simulink model "car_model_FIXED"  (R2022b)
settings: Solver=VariableStepAuto  StartTime=0.0  StopTime=60  RelTol=1e-3
values from neighbouring files (symbols this model uses):
  ABS_MAX_TORQUE = [25 25 25 25]    [Startup.m]
  ABS_MAX_TRQ_CMD = dot(ABS_MAX_TORQUE, MOTOR_ENABLE)    [Startup.m]
  ABS_MIN_TORQUE = [0.01 0.01 0.01 0.01]    [Startup.m]
  acc_IC = 0    [Startup.m]
  ACCELERATION_MAX = 30    [Startup.m]
  ang_IC = 0    [Startup.m]
  ang_vel_IC = 0    [Startup.m]
  ax = Reference_Signals.Chassis_Acceleration_VNED.ax.Data(:)    [Simulation_Data_Parse.m]    (also in Vehicle_Sim_Parse.m)
  ay = Reference_Signals.Chassis_Acceleration_VNED.ay.Data(:)    [Simulation_Data_Parse.m]    (also in Vehicle_Sim_Parse.m)
  az = Reference_Signals.Chassis_Acceleration_VNED.az.Data(:)    [Simulation_Data_Parse.m]    (also in Vehicle_Sim_Parse.m)
  battery_current_IC = 0    [Startup.m]
  BATTERY_CURRENT_MAX = 140    [Startup.m]
  BATTERY_CURRENT_MIN = 0    [Startup.m]
  battery_FT_IC = 300    [Startup.m]
  battery_T_IC = 300    [Startup.m]
  BATTERY_TEMPERATURE_MAX = 60    [Startup.m]
  BATTERY_TEMPERATURE_MIN = 0    [Startup.m]
  battery_voltage_IC = Ns*max(Em)    [Startup.m]
  BATTERY_VOLTAGE_MAX = 340    [Startup.m]
  BATTERY_VOLTAGE_MIN = 60    [Startup.m]
  Brake_Pressure_IC = 1    [Startup.m]
  ccl_IC = 0    [Startup.m]
  CENTER_STEER_ANGLE_MAX = 130    [Startup.m]
  covarience_matrix_IC = Simulink.Parameter(eye(28)./1000)    [Startup.m]
  dcl_IC = 140    [Startup.m]
  DCL_MAX = 130    [Startup.m]
  DCL_MIN = 0    [Startup.m]
  driver_t = 0.015    [Startup.m]
  fusion_t = Simulink.Parameter(0.01)    [Startup.m]
  fusion_t_sim = fusion_t.copy    [Startup.m]
  Fz_IC = m_all*g/4    [Startup.m]
  g = 9.81    [Startup.m]
  gps_hz = 0.01    [Startup.m]
  gps_ratio = Simulink.Parameter(gps_hz / imu_hz.Value)    [Startup.m]
  imu_hz = fusion_t.copy    [Startup.m]
  location_lla_IC = Simulink.Parameter([40.437675, -86.943750, 200])    [Startup.m]
  MAG_MAX = 200    [Startup.m]
  Max_Brake_Pressure = 10^8    (= 100000000)    [Startup.m]
  Max_Driver_Input = 1    [Startup.m]
  MAX_DTHETA_DRIVER = 360    [Startup.m]
  MAX_STEERING_ADJUST = 15    [Startup.m]
  Min_Brake_Pressure = 1    [Startup.m]
  Min_Driver_Input = 0    [Startup.m]
  motor_current_IC = 0    [Startup.m]
  MOTOR_CURRENT_MAX = 70    [Startup.m]
  MOTOR_CURRENT_MIN = 0    [Startup.m]
  MOTOR_ENABLE = [0 0 1 1]    [Startup.m]
  motor_FT_IC = 300    [Startup.m]
  motor_T_IC = 300    [Startup.m]
  MOTOR_TEMPERATURE_MAX = 100    [Startup.m]
  MOTOR_TEMPERATURE_MIN = 0    [Startup.m]
  motor_voltage_IC = 332    [Startup.m]
  MOTOR_VOLTAGE_MAX = 340    [Startup.m]
  MOTOR_VOLTAGE_MIN = 90    [Startup.m]
  omega_IC = 0    [Startup.m]
  OMEGA_MAX = 150    [Startup.m]
  OMEGA_MIN = 0    [Startup.m]
  ORIENTATION_MAX = 360    [Startup.m]
  pos_IC = 0    [Startup.m]
  POS_MAX = 300    [Startup.m]
  rho = 1.225    [Startup.m]
  selected_maxvm = MIN_TRACK_DATA.(event_names(10))    [Startup.m]
  selected_sweep = ALL_SWEEP_DATA.(sweep_names(1))    [Startup.m]
  selected_track = ALL_TRACK_DATA.(event_names(10))    [Startup.m]
  shock_length_IC = 0.1    [Startup.m]
  SHOCK_LENGTH_MAX = 0.25    [Startup.m]
  SHOCK_LENGTH_MIN = 0    [Startup.m]
  state_IC = zeros(28,1)    [Startup.m]
  theta_IC = 0    [Startup.m]
  TRACTION_ENABLE = 0    [Startup.m]
  TVS_ENABLE = 0    [Startup.m]
  tvs_t = 0.015    [Startup.m]
  tvs_t_sim = tvs_t    (= 0.015)    [Startup.m]
  Tx_I = 0    [Startup.m]
  vel_IC = [0 0 0]    [Startup.m]
  VELOCITY_MAX = 30    [Startup.m]
  X = Reference_Signals.Chassis_Position.X.Data(:)    [Simulation_Data_Parse.m]    (also in Vehicle_Sim_Parse.m = Chassis_Signals.InertFrm.Cg.Disp.X.Data(:))
  Y = Reference_Signals.Chassis_Position.Y.Data(:)    [Simulation_Data_Parse.m]    (also in Vehicle_Sim_Parse.m = Chassis_Signals.InertFrm.Cg.Disp.Y.Data(:))
  YAW_ENABLE = 1    [Startup.m]
  YAW_MAX = 2.5    [Startup.m]
undefined symbols (not defined in the file or in its folder): ActSuspDutyCycle, Aeq_left, Aeq_right, alpha_error, ang_acc_hystersesis, area_air, axb, br, brake_bias, covA, covG, covM, covP, covV, CURRENT_BUFFER, cy_sweep, dB, deadband_angle, dIndex, DiscIntNeverNeededParam, dt_OFF, dt_ON, dTx, dx, dZ, efficiency_grid, F0z, forward_look_straight, forward_look_turn, Fz_sweep, GAIN_ABS, gearbox_efficiency, gr, I, I_Driver, IMU_accel, IMU_gyro, IMU_mag, IMUNED2VNED, indicies, IYY, kx_sweep, l, lambda_star, low_V_SA, lr, m_all, m_body, m_unsprung, MAGNED2VNED, MAX_I_Driver, max_yaw, min_velocity_regen, motorControllerCurve, motorTempCurve, motorTempX, mu_star, mx_sweep, my_sweep, noise_state ... (+40)
libraries: fl_lib x82, nesl_utility x32, vehdynlibtire x10, vehdynlibsuspension x8, simulink x5, autolibutils x5, sharedtransform x5, sdl_lib x4, EngineCoolingComponents_lib x4, slpidlib x3, SimscapeFluids_lib x3, shared6dof x2
(part 5 of 14)

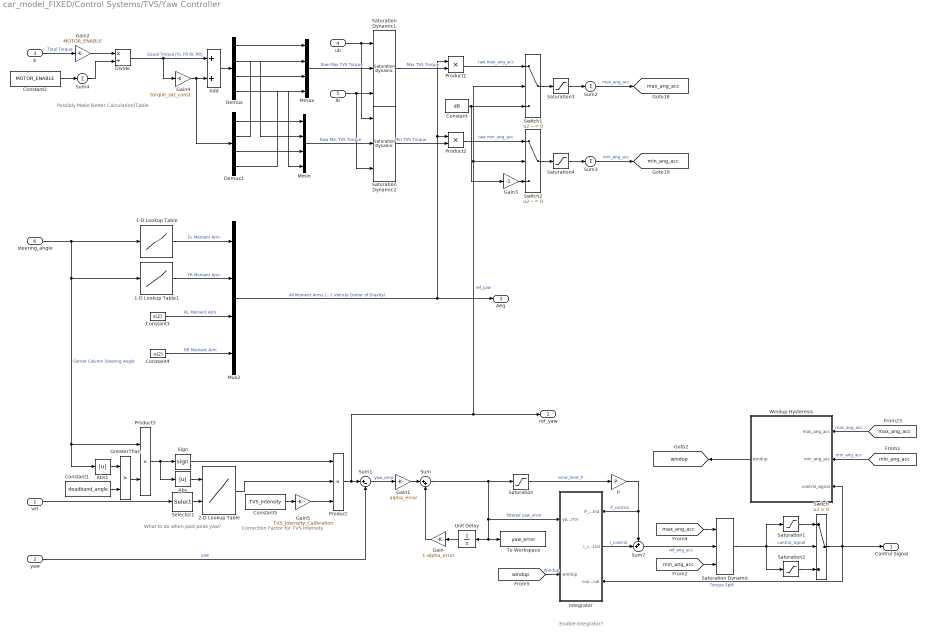
== system car_model_FIXED/Control Systems/TVS/Yaw Controller ==
  note: Correction Factor for TVS Intensity
  note: Enable Integrator?
  note: What to do when past peak yaw?
  note: Possibly Make Better Calculation/Table
  vel : Inport
  yaw : Inport  Port=2  OutDataTypeStr=double  LockScale=on
  b : Inport  Port=3
  ub : Inport  Port=4
  lb : Inport  Port=5
  steering_angle : Inport  Port=6
  1-D Lookup Table : Lookup_n-D  NumberOfTableDimensions=1  BreakpointsForDimension1=theta_sweep  Table=Aeq_left  ExtrapMethod=Clip  InternalRulePriority=Speed  RndMeth=Simplest
  1-D Lookup Table1 : Lookup_n-D  NumberOfTableDimensions=1  BreakpointsForDimension1=theta_sweep  Table=Aeq_right  ExtrapMethod=Clip  InternalRulePriority=Speed  RndMeth=Simplest
  2-D Lookup Table : Lookup_n-D  BreakpointsForDimension1=steering_sweep  BreakpointsForDimension2=velocity_sweep  Table=yaw_rate  ExtrapMethod=Clip  InternalRulePriority=Speed  RndMeth=Simplest
      settings: InputPortMap=u0,u1
  Abs : Abs  SaturateOnIntegerOverflow=off
  Abs1 : Abs  SaturateOnIntegerOverflow=off
  Add : Sum
  Constant : Constant  Value=dB  OutDataTypeStr=Inherit: Inherit via back propagation
  Constant1 : Constant  Value=deadband_angle
  Constant2 : Constant  Value=MOTOR_ENABLE
  Constant3 : Constant  Value=s(2)  OutDataTypeStr=Inherit: Inherit via back propagation
  Constant4 : Constant  Value=-s(2)  OutDataTypeStr=Inherit: Inherit via back propagation
  Constant5 : Constant  Value=TVS_Intensity
  Demux : Demux
  Demux1 : Demux
  Divide : Product  Inputs=*/
  Gain : Gain  Gain=1-alpha_error
  Gain1 : Gain  Gain=alpha_error
  Gain2 : Gain  Gain=MOTOR_ENABLE
  Gain3 : Gain  Gain=-1
  Gain4 : Gain  Gain=torque_sat_const
  Gain5 : Gain  Gain=TVS_Intensity_Calibration
  GreaterThan : RelationalOperator  Operator=>  OutDataTypeStr=boolean  RndMeth=Simplest  InputSameDT=off
  Integrator : Subsystem
      settings: PortSchema="{\"entries\":[{\"content\":{\"sides\":[{\"content\":{\"connectorIds\":[\"In1\",\"In2\"]},\"type\":\"ConnectorPlacement.EquallySpacedRectSide\",\"uuid\":\"8eceed30-5463-482b-9ad9-1d0859eec1e0\"},{\"content\":{\"connectorIds\":[\"In3\",\"Out1\",\"In4\"],\"side\":\"RIGHT\"},\"type\":\"ConnectorPlacement.EquallySpacedRectSide\",\"uuid\":\"ca18b8b2-b2b4-4da4-8362-ca68ae703b33\"},{\"content\":{\"connectorIds\":[],\"side\":\"TOP\"},\"type\":\"ConnectorPlacement.EquallySpacedRectSide\",\"uuid\":\"14e81d29-e47e-408e-961b-b14eadc3d40e\"}]},\"type\":\"ConnectorPlacement.EquallySpacedConnector\",\"uuid\":\"147d3fcd-d0df-4d8b-910b-d1c7e2c77e1f\"}],\"packageUris\":[\"http://schema.mathworks.com/mf0/Connector/R2020b\"],\"version\":\"1.0\"}"
  Mmax : Mux
  Mmin : Mux
  Mux2 : Mux
  P : Gain  Gain=P  ParamDataTypeStr=double  OutDataTypeStr=double
  Product : Product  Inputs=3  OutDataTypeStr=Inherit: Inherit via back propagation
  Product1 : Product
  Product2 : Product
  Product3 : Product
  Saturation : Saturate  UpperLimit=YAW_MAX  LowerLimit=-YAW_MAX
  Saturation Dynamic : simulink/Discontinuities/Saturation Dynamic  OutMin=[]  OutMax=[]  OutDataTypeStr=Inherit: Same as second input  OutDataType=fixdt(1, 16)  OutScaling=2^-10  DoSatur=off
  Saturation Dynamic1 : simulink/Discontinuities/Saturation Dynamic  OutMin=[]  OutMax=[]  OutDataTypeStr=Inherit: Same as second input  OutDataType=fixdt(1, 16)  OutScaling=2^-10  DoSatur=off
  Saturation Dynamic2 : simulink/Discontinuities/Saturation Dynamic  OutMin=[]  OutMax=[]  OutDataTypeStr=Inherit: Same as second input  OutDataType=fixdt(1, 16)  OutScaling=2^-10  DoSatur=off
  Saturation1 : Saturate  UpperLimit=inf  LowerLimit=dB
  Saturation2 : Saturate  UpperLimit=-dB  LowerLimit=-inf
  Saturation3 : Saturate  UpperLimit=inf  LowerLimit=dB
  Saturation4 : Saturate  UpperLimit=-dB  LowerLimit=-inf
  Selector1 : Selector  InputPortWidth=4  IndexOptions=Index vector (dialog)  Indices=4  OutputSizes=1
  Sign : Signum
  Sum : Sum  Inputs=|++
  Sum1 : Sum  Inputs=|+-  OutDataTypeStr=Inherit: Inherit via back propagation
  Sum2 : Sum  Inputs=+
  Sum3 : Sum  Inputs=+
  Sum4 : Sum  Inputs=+
  Sum7 : Sum  Inputs=++|  OutDataTypeStr=double  SaturateOnIntegerOverflow=on
  Switch : Switch  Criteria=u2 > Threshold  SaturateOnIntegerOverflow=off  InputSameDT=off
  Switch1 : Switch  Criteria=u2 ~= 0  OutDataTypeStr=Inherit: Inherit via back propagation  SaturateOnIntegerOverflow=off  InputSameDT=off
  Switch2 : Switch  Criteria=u2 ~= 0  OutDataTypeStr=Inherit: Inherit via back propagation  SaturateOnIntegerOverflow=off  InputSameDT=off
  To Workspace : ToWorkspace  VariableName=yaw_error  SaveFormat=Timeseries  SampleTime=-1
  Unit Delay : UnitDelay  SampleTime=-1  HasFrameUpgradeWarning=on
  Windup Hysteresis : Subsystem
  Control Signal : Outport  OutDataTypeStr=double  PortDimensions=1  LockScale=on
  ref_yaw : Outport  Port=2
  Aeq : Outport  Port=3  OutDataTypeStr=double  LockScale=on
  tag scope: max_ang_acc=global, min_ang_acc=global, windup=global
  wires:
  P/1 -> Sum7/1, Integrator/3(P_control)  "P_control"
  yaw/1 -> Sum1/2  "yaw"
  Integrator/1(I_control) -> Sum7/2  "I_control"
  Sum7/1 -> Saturation Dynamic/2  "ref_ang_acc"
  Saturation Dynamic/1 -> Saturation2/1, Saturation1/1, Switch/2  "control_signal"
  Sum2/1 -> [max_ang_acc]  "max_ang_acc"
  Sum3/1 -> [min_ang_acc]  "min_ang_acc"
  Saturation/1 -> P/1  "error_limit_P"
  Windup Hysteresis/1(windup) -> [windup]
  Sum/1 -> Saturation/1, Unit Delay/1, To Workspace/1, Integrator/1(yaw_error)  "filtered yaw_error"
  [windup] -> Integrator/2(windup)  "Windup"
  Unit Delay/1 -> Gain/1
  Gain/1 -> Sum/2
  Gain1/1 -> Sum/1
  Sum1/1 -> Gain1/1  "yaw_error"
  Switch/1 -> Windup Hysteresis/3(control_signal), Control Signal/1, Integrator/4(control_signal)  "Torque Split"
  Saturation1/1 -> Switch/1
  Saturation2/1 -> Switch/3
  Saturation4/1 -> Sum3/1
  Gain3/1 -> Switch2/3
  Demux1/4 -> Mmax/4
  Constant4/1 -> Mux2/4  "RR Moment Arm"
  Switch2/1 -> Saturation4/1
  b/1 -> Gain2/1  "Total Torque"
  Constant3/1 -> Mux2/3  "RL Moment Arm"
  1-D Lookup Table/1 -> Mux2/1  "FL Moment Arm"
  Demux/3 -> Mmax/3
  Gain4/1 -> Demux1/1, Add/2
  Demux1/3 -> Mmin/3
  Product1/1 -> Switch1/1  "raw max_ang_acc"
  Demux/4 -> Mmin/4
  1-D Lookup Table1/1 -> Mux2/2  "FR Moment Arm"
  Demux/2 -> Mmin/2
  Mux2/1 -> Aeq/1, Product2/1, Product1/1  "All Moment Arms {FL FR RL RR] (about Vehicle Center of Gravity)"
  Demux/1 -> Mmax/1
  Add/1 -> Demux/1
  Demux1/2 -> Mmax/2
  ub/1 -> Saturation Dynamic2/1, Saturation Dynamic1/1
  Saturation Dynamic1/1 -> Product1/2  "Max TVS Torque"
  Demux1/1 -> Mmin/1
  lb/1 -> Saturation Dynamic2/3, Saturation Dynamic1/3
  Product2/1 -> Switch2/1  "raw min_ang_acc"
  Mmax/1 -> Saturation Dynamic1/2  "Raw Max TVS Torque"
  Constant/1 -> Switch1/3, Gain3/1
  Saturation3/1 -> Sum2/1
  Mmin/1 -> Saturation Dynamic2/2  "Raw Min TVS Torque"
  Saturation Dynamic2/1 -> Product2/2  "Min TVS Torque"
  Divide/1 -> Gain4/1, Add/1  "Equal Torque [FL FR RL RR]"
  Switch1/1 -> Saturation3/1
  Product/1 -> ref_yaw/1, Switch2/2, Switch1/2, Sum1/1  "ref_yaw"
  Constant1/1 -> GreaterThan/2
  steering_angle/1 -> 1-D Lookup Table1/1, Abs1/1, Product3/1, 1-D Lookup Table/1  "Center Column Steering Angle"
  vel/1 -> Selector1/1
  Abs/1 -> 2-D Lookup Table/1
  Product3/1 -> Abs/1, Sign/1
  Sign/1 -> Product/1
  Abs1/1 -> GreaterThan/1
  GreaterThan/1 -> Product3/2
  Selector1/1 -> 2-D Lookup Table/2
  [min_ang_acc] -> Windup Hysteresis/2(min_ang_acc)  "min_ang_acc"
  [max_ang_acc] -> Windup Hysteresis/1(max_ang_acc)  "max_ang_acc"
  [min_ang_acc] -> Saturation Dynamic/3
  [max_ang_acc] -> Saturation Dynamic/1
  Constant5/1 -> Gain5/1
  2-D Lookup Table/1 -> Product/2
  Gain5/1 -> Product/3
  Constant2/1 -> Sum4/1
  Gain2/1 -> Divide/1
  Sum4/1 -> Divide/2

== system car_model_FIXED/Driver & Environment/Longitudinal Control/AAS ==
  v_error : Inport
  Abs : Abs  SaturateOnIntegerOverflow=off
  Constant : Constant
  Discrete-Time Integrator : DiscreteIntegrator  ExternalReset=rising  SampleTime=-1  LimitOutput=on  UpperSaturationLimit=MAX_I_Driver  LowerSaturationLimit=-MAX_I_Driver  ICPrevOutput=DiscIntNeverNeededParam  ICPrevScaledInput=DiscIntNeverNeededParam
  Gain : Gain  Gain=P_Driver
  Gain1 : Gain  Gain=I_Driver
  Less Than : RelationalOperator  Operator=<  OutDataTypeStr=boolean  RndMeth=Simplest  InputSameDT=off
  NOT : Logic  Operator=NOT  IconShape=distinctive  AllPortsSameDT=off  OutDataTypeStr=boolean
  Product : Product
  Saturation : Saturate  UpperLimit=Max_Driver_Input  LowerLimit=Min_Driver_Input
  Sum2 : Sum  Inputs=|++
  driver_input : Outport
  wires:
  Constant/1 -> Less Than/2
  Gain1/1 -> Discrete-Time Integrator/1
  Gain/1 -> Sum2/1
  Sum2/1 -> Saturation/1
  Discrete-Time Integrator/1 -> Sum2/2
  Less Than/1 -> NOT/1, Product/2
  NOT/1 -> Discrete-Time Integrator/2
  Abs/1 -> Less Than/1
  Product/1 -> Gain1/1
  Saturation/1 -> driver_input/1
  v_error/1 -> Abs/1, Product/1, Gain/1  "v_error"

== system car_model_FIXED/Driver & Environment/Longitudinal Control/ABS ==
  Vx : Inport
  omega : Inport  Port=2
  ABS_ENABLE : Inport  Port=3
  ABS system : Subsystem
  Extremum Seeking Control : slctrlblks/Extremum Seeking Control  timeDomainStatus=Discrete time  SampleTime=driver_t  IntegratorMethods=Backward Euler  paramCount=N  initialVal=IC  omega=omega_force  gain=lr  demodAmp=a  demodPhase=phi_1  modAmp=b  modPhase=phi_2  highPassEnable=on  highPassCutoff=omega_hpf  lowPassEnable=on  lowPassCutoff=omega_lpf  estimatedVarOn=off  HPFFreq=-0.99253  LPFFreq=-0.98511  SampleTimeVar=0.015
  Gain6 : Gain  Gain=GAIN_ABS*brake_bias
  Sum : Sum  Inputs=+
  Unit Delay : UnitDelay  SampleTime=-1  HasFrameUpgradeWarning=on
  Bx : Outport
  OFF_FLAG : Outport  Port=2
  wires:
  ABS system/1(mu) -> Unit Delay/1
  Extremum Seeking Control/1 -> ABS system/1(lambda0)
  Vx/1 -> ABS system/2(Vx)
  omega/1 -> ABS system/3(omega)
  ABS system/3(OFF_FLAG) -> OFF_FLAG/1
  ABS system/2(Bx) -> Sum/1
  ABS_ENABLE/1 -> ABS system/4(ABS_ENABLE)
  Sum/1 -> Gain6/1
  Gain6/1 -> Bx/1
  Unit Delay/1 -> Extremum Seeking Control/1

== system car_model_FIXED/Driver & Environment/Reference Generator/Subsystem ==
  <psi> : Inport
  Constant1 : Constant  Value=2*pi
  Constant2 : Constant  Value=pi
  Constant3 : Constant  Value=-pi
  Constant4 : Constant  Value=2*pi
  Constant5 : Constant  Value=-2*pi
  GreaterThan : RelationalOperator  Operator=>  OutDataTypeStr=boolean  RndMeth=Simplest  InputSameDT=off
  Less Than : RelationalOperator  Operator=<  OutDataTypeStr=boolean  RndMeth=Simplest  InputSameDT=off
  Mod : Math  Operator=mod
  Product : Product
  Product1 : Product
  Sum : Sum  Inputs=+++
  psi_rev : Outport
  wires:
  Product1/1 -> Sum/3
  Less Than/1 -> Product1/2
  GreaterThan/1 -> Product/1
  Mod/1 -> GreaterThan/1, Sum/1, Less Than/1
  Constant1/1 -> Mod/2
  Constant5/1 -> Product/2
  Constant3/1 -> Less Than/2
  Constant4/1 -> Product1/1
  Constant2/1 -> GreaterThan/2
  Product/1 -> Sum/2
  Sum/1 -> psi_rev/1
  <psi>/1 -> Mod/1

== system car_model_FIXED/Vehicle Model/Electronics/360_180 ==
  <psi> : Inport
  Constant1 : Constant  Value=2*pi
  Constant2 : Constant  Value=pi
  Constant3 : Constant  Value=-pi
  Constant4 : Constant  Value=2*pi
  Constant5 : Constant  Value=-2*pi
  GreaterThan : RelationalOperator  Operator=>  OutDataTypeStr=boolean  RndMeth=Simplest  InputSameDT=off
  Less Than : RelationalOperator  Operator=<  OutDataTypeStr=boolean  RndMeth=Simplest  InputSameDT=off
  Mod : Math  Operator=mod
  Product : Product
  Product1 : Product
  Sum : Sum  Inputs=+++
  psi_rev : Outport
  wires:
  Product1/1 -> Sum/3
  Less Than/1 -> Product1/2
  GreaterThan/1 -> Product/1
  Mod/1 -> GreaterThan/1, Sum/1, Less Than/1
  Constant1/1 -> Mod/2
  Constant5/1 -> Product/2
  Constant3/1 -> Less Than/2
  Constant4/1 -> Product1/1
  Constant2/1 -> GreaterThan/2
  Product/1 -> Sum/2
  Sum/1 -> psi_rev/1
  <psi>/1 -> Mod/1

== system car_model_FIXED/Vehicle Model/Electronics/Cooling Sensors ==
  <motor_temperature> : Inport
  <mc_temp> : Inport  Port=2
  <motor_fluid_temperature> : Inport  Port=3
  <battery_temperature> : Inport  Port=4
  <battery_fluid_temperature> : Inport  Port=5
  motor_temperature : Outport
  mc_temp : Outport  Port=2
  motor_fluid_temperature : Outport  Port=3
  battery_temperature : Outport  Port=4
  battery_fluid_temperature : Outport  Port=5
  wires:
  <motor_temperature>/1 -> motor_temperature/1
  <motor_fluid_temperature>/1 -> motor_fluid_temperature/1
  <battery_temperature>/1 -> battery_temperature/1
  <battery_fluid_temperature>/1 -> battery_fluid_temperature/1
  <mc_temp>/1 -> mc_temp/1

== system car_model_FIXED/Vehicle Model/Electronics/Corner Dynamics Sensors ==
  <omega> : Inport
  <steering_angle> : Inport  Port=2
  <shock_length> : Inport  Port=3
  <Fz> : Inport  Port=4
  Transpose : Math  Operator=transpose
  omega : Outport
  steering_angle : Outport  Port=2
  shock_length : Outport  Port=3
  Fz : Outport  Port=4
  wires:
  Transpose/1 -> omega/1  "omega"
  <omega>/1 -> Transpose/1
  <steering_angle>/1 -> steering_angle/1
  <shock_length>/1 -> shock_length/1
  <Fz>/1 -> Fz/1

== system car_model_FIXED/Vehicle Model/Electronics/Navigation Sensors ==
  <chassis_velocity> : Inport  PortDimensions=[1 3]
  <chassis_position> : Inport  Port=2  PortDimensions=[1 3]
  <chassis_acceleration> : Inport  Port=3  PortDimensions=[1 3]
  <chassis_orientation> : Inport  Port=4  PortDimensions=[1 3]
  <chassis_angular_velocity> : Inport  Port=5  PortDimensions=[1 3]
  Bus Creator : BusCreator  Inputs=IMU_accel,IMU_gyro,IMU_mag
  Bus Creator1 : BusCreator  Inputs=2
  GPS : sensorgpslib/GPS  DispRefFrame=NED  PositionInputFormat=Local  ReferenceLocation=location_lla_IC  HorizontalPositionAccuracy=GPS_Z_ACCURACY  VerticalPositionAccuracy=GPS_XY_ACCURACY  VelocityAccuracy=GPS_V_ACCURACY  DecayFactor=GPS_NOISE_FACTOR  SeedDouble=r_GPS  SimulateUsing=Interpreted execution
      settings: LibrarySourceBlock=mspsensorlib/GPS
  IMU : mspsensorlib/IMU  DispRefFrame=NED  Temperature=25  MagneticFieldNED=mag_field_IC  MagneticFieldENU=[ -2.4169, 27.5550, 16.0849 ]  SeedDouble=r_IMU  SimulateUsing=Interpreted execution  AccelParamsMeasurementRange=ACC_MAX  AccelParamsResolution=ACC_RES  AccelParamsConstantBias=ACC_BIAS  AccelParamsAxesMisalignment=ACC_SKEW  AccelParamsNoiseDensity=ACC_VEL_WALK  AccelParamsBiasInstability=ACC_BIAS_INSTABILITY  AccelParamsRandomWalk=ACC_WALK  AccelParamsTemperatureBias=ACC_T_BIAS  AccelParamsTemperatureScaleFactor=ACC_T_SCALE  GyroParamsMeasurementRange=GYR_MAX  GyroParamsResolution=GYR_RES  GyroParamsConstantBias=GYR_BIAS  GyroParamsAxesMisalignment=GYR_SKEW  GyroParamsAccelerationBias=GYR_ACC_BIAS  GyroParamsNoiseDensity=GYR_ANG_WALK  GyroParamsBiasInstability=GYR_BIAS_INSTABILITY  GyroParamsRandomWalk=GYR_WALK  GyroParamsTemperatureBias=GYR_T_BIAS  GyroParamsTemperatureScaleFactor=GYR_T_SCALE  MagParamsMeasurementRange=MAG_MAX  MagParamsResolution=MAG_RES  MagParamsConstantBias=MAG_BIAS  MagParamsAxesMisalignment=MAG_SKEW  MagParamsNoiseDensity=MAG_WHITE  MagParamsBiasInstability=MAG_BIAS_INSTABILITY  MagParamsRandomWalk=MAG_WALK  MagParamsTemperatureBias=MAG_T_BIAS  MagParamsTemperatureScaleFactor=MAG_T_SCALE
  To Workspace1 : ToWorkspace  VariableName=Chassis_Orientation  SaveFormat=Timeseries  SampleTime=-1
  To Workspace2 : ToWorkspace  VariableName=IMU_Measurements  SaveFormat=Timeseries  SampleTime=-1
  Transpose : Math  Operator=transpose
  Transpose1 : Math  Operator=transpose
  Transpose2 : Math  Operator=transpose
  VNED to SNED : MATLAB Function  TreatAsAtomicUnit=on
  integrate angvel : MATLAB Function  TreatAsAtomicUnit=on
  vel : Outport  PortDimensions=3
  pos : Outport  Port=2  PortDimensions=3
  acc : Outport  Port=3  PortDimensions=3
  mag : Outport  Port=4  PortDimensions=3
  gyro : Outport  Port=5  PortDimensions=3
  GS : Outport  Port=6
  Course : Outport  Port=7
  wires:
  <chassis_angular_velocity>/1 -> IMU/2  "ang_vel_VNED"
  <chassis_velocity>/1 -> GPS/2  "vel_NED"
  <chassis_acceleration>/1 -> IMU/1  "accel_VNED"
  <chassis_position>/1 -> GPS/1  "pos_NED"
  integrate angvel/1(Orientation_c) -> Bus Creator1/1, IMU/3  "ang_NED"
  GPS/4 -> Course/1  "ang_NE_mag"
  GPS/3 -> GS/1  "vel_NE_mag"
  GPS/2 -> vel/1  "vel_NED"
  GPS/1 -> pos/1  "pos_LLA"
  VNED to SNED/2(gyro_SNED) -> gyro/1  "gyro_SNED"
  VNED to SNED/1(accel_SNED) -> acc/1  "accel_SNED"
  VNED to SNED/3(mag_SNED) -> mag/1  "mag_SNED"
  <chassis_orientation>/1 -> integrate angvel/1("Orientation_e ")  "ang_NED"
  Transpose2/1 -> Bus Creator/3, VNED to SNED/3(mag_VNED)  "IMU_mag"
  Transpose1/1 -> Bus Creator/2, VNED to SNED/2(gyro_VNED)  "IMU_gyro"
  Transpose/1 -> Bus Creator/1, VNED to SNED/1(accel_VNED)  "IMU_accel"
  IMU/3 -> Transpose2/1
  IMU/1 -> Transpose/1
  IMU/2 -> Transpose1/1
  Bus Creator/1 -> To Workspace2/1
  Bus Creator1/1 -> To Workspace1/1
  integrate angvel/2(Orientation_e) -> Bus Creator1/2  "ang_euler_NED"

== system car_model_FIXED/Vehicle Model/Electronics/Power Sensors ==
  <battery_voltage> : Inport
  <battery_current> : Inport  Port=2
  <motor_voltage> : Inport  Port=3
  <motor_current> : Inport  Port=4
  <power_limits> : Inport  Port=5
  battery_voltage : Outport
  battery_current : Outport  Port=2
  motor_voltage : Outport  Port=3
  motor_current : Outport  Port=4
  power_limits : Outport  Port=5
  wires:
  <battery_voltage>/1 -> battery_voltage/1
  <battery_current>/1 -> battery_current/1
  <motor_voltage>/1 -> motor_voltage/1
  <power_limits>/1 -> power_limits/1
  <motor_current>/1 -> motor_current/1

== system car_model_FIXED/Vehicle Model/Powertrain/Battery Cooling Loop ==
  omega_m : Inport
  Battery_V : Inport  Port=2
  Battery_I : Inport  Port=3
  CL Battery Fans : Inport  Port=4
  CL Battery Pump : Inport  Port=5
  Vg : Inport  Port=6
  Battery Temperature : Outport
  Battery Fluid Temperature : Outport  Port=2

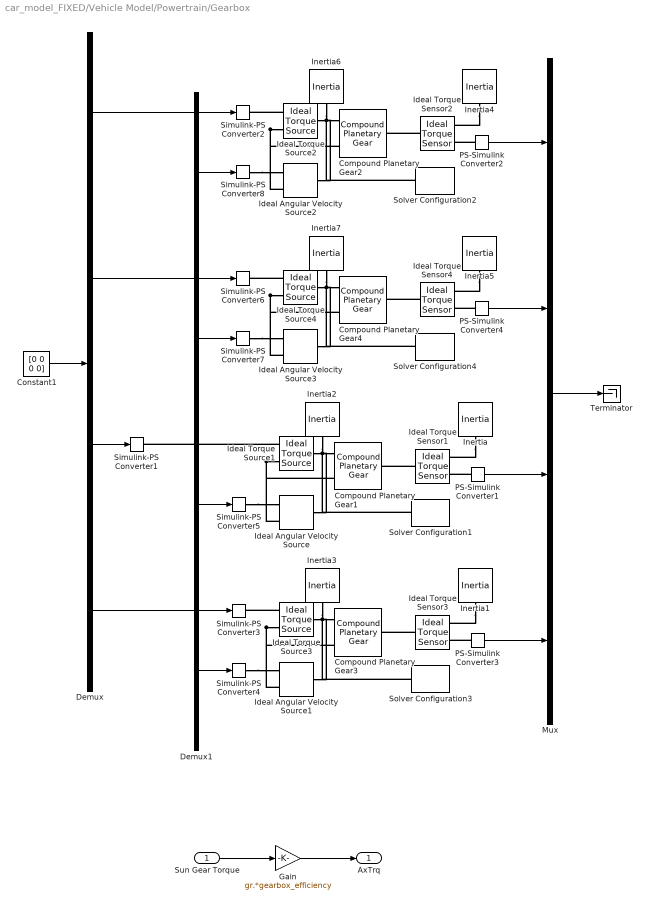
== system car_model_FIXED/Vehicle Model/Powertrain/Gearbox ==
  Sun Gear Torque : Inport
  Compound Planetary Gear{1..4} (4 alike) : sdl_lib/Gears/Compound Planetary Gear  rp_ratio=84/23  ps_ratio=40/21  friction_model=sdl.enum.gear_friction.constant  efficiency=[.97, 1]  temperature_TLU=[280, 300, 320] K  efficiency_sp_TLU=[.95, .9, .85]  efficiency_rp_TLU=[.95, .9, .85]  pwr_thr=[.001, .001] W  mu_visc=[0, 0] N*m/(rad/s)  model_inertia=simscape.enum.onoff.on  planet_inertia=0.001 kg*m^2  thermal_mass=50 J/K  T_init=300 K
      settings: InternalSimscapePortConfiguration="{\"Bottom\":[],\"Left\":[{\"id\":\"C\",\"label\":\"C\",\"type\":\"foundation.mechanical.rotational.rotational\"}],\"Right\":[{\"id\":\"R\",\"label\":\"R\",\"type\":\"foundation.mechanical.rotational.rotational\"},{\"id\":\"S\",\"label\":\"S\",\"type\":\"foundation.mechanical.rotational.rotational\"}],\"Top\":[]}"
  Constant1 : Constant  Value=[0 0 0 0]
  Demux : Demux
  Demux1 : Demux
  Gain : Gain  Gain=gr.*gearbox_efficiency
  Ideal Angular Velocity Source{,1..3} (4 alike) : fl_lib/Mechanical/Mechanical Sources/Ideal Angular Velocity Source
  Ideal Torque Sensor{1..4} (4 alike) : fl_lib/Mechanical/Mechanical Sensors/Ideal Torque Sensor
  Ideal Torque Source{1..4} (4 alike) : fl_lib/Mechanical/Mechanical Sources/Ideal Torque Source
  Inertia{,1,4..5} (4 alike) : fl_lib/Mechanical/Rotational Elements/Inertia  inertia=0.01 kg*m^2  num_ports=foundation.enum.numPorts2.one  w_specify=off  w_priority=High  w=0 rad/s  w_nominal_specify=off  w_nominal_unit=rad/s  w_nominal_value=1  t_specify=off  t_priority=None  t=0 N*m  t_nominal_specify=off  t_nominal_unit=N*m  t_nominal_value=1
  Inertia{2..3,6..7} (4 alike) : fl_lib/Mechanical/Rotational Elements/Inertia  inertia=0.01 kg*m^2  num_ports=foundation.enum.numPorts2.one  w_specify=off  w_priority=High  w=0 rad/s  w_nominal_specify=off  w_nominal_unit=rad/s  w_nominal_value=1  t_specify=on  t_priority=High  t=0 N*m  t_nominal_specify=off  t_nominal_unit=N*m  t_nominal_value=1
  Mux : Mux
  PS-Simulink Converter{1..4} (4 alike) : nesl_utility/PS-Simulink Converter  PhysicalDomain=network_engine_domain  SubClassName=ps_output  LeftPortType=input  RightPortType=output  PseudoPeriodic=off  Frequencies=[]  VectorFormat=1-D array  Unit=inherit  AffineConversion=off
  Simulink-PS Converter{1..3,6} (4 alike) : nesl_utility/Simulink-PS Converter  PhysicalDomain=network_engine_domain  SubClassName=ps_input  LeftPortType=input  RightPortType=output  PseudoPeriodic=off  Frequencies=[]  NoiseDistribution=none  NoiseParameters=[]  Unit=N*m  AffineConversion=off  FilteringAndDerivatives=zero  SimscapeFilterOrder=1  InputFilterTimeConstant=0.001  UdotUserProvided=0
  Simulink-PS Converter{4..5,7..8} (4 alike) : nesl_utility/Simulink-PS Converter  PhysicalDomain=network_engine_domain  SubClassName=ps_input  LeftPortType=input  RightPortType=output  PseudoPeriodic=off  Frequencies=[]  NoiseDistribution=none  NoiseParameters=[]  Unit=rad/s  AffineConversion=off  FilteringAndDerivatives=zero  SimscapeFilterOrder=1  InputFilterTimeConstant=0.001  UdotUserProvided=0
  Solver Configuration{1..4} (4 alike) : nesl_utility/Solver Configuration  PhysicalDomain=network_engine_domain  SubClassName=solver  LeftPortType=input  RightPortType=generic  Tones=[]  Harmonics=[]  SimulateNoise=off  Profile=off  UseLocalSampling=off  EnableSwitchedLinearOptims=on  FrequencyDomain=off  UseCCode=off  RelTol=0.001  AbsTol=1e-06  MinStep=1e-09  ToWorkspace=off  RevertToSquareIcSolve=off  NumHomotopyIterations=100  PhasorMode=off  PhasorModeNumHarmonics=1  ConsistencySolver=NEWTON_FTOL  IndexReductionMethod=DerivativeReplacement  DoDC=off  ResidualTolerance=1e-09  ConsistencyTolSource=GLOBAL  ConsistencyAbsTol=0.001  ConsistencyRelTol=0.001  ConsistencyTolFactor=0.001  UseLocalSolver=off  LocalSolverChoice=NE_BACKWARD_EULER_ADVANCER  ResolveIndetEquations=on  FunctionEvalNumThread=1  LocalSolverSampleTime=0.000001  DoFixedCost=off  MaxNonlinIter=300  MaxModeIter=2  ComputeImpulses=off  ImpulseIterations=2  LinearAlgebra=auto  LinearAlgebraNumThread=0  EquationFormulation=NE_TIME_EF  DelaysMemoryBudget=1024  AutomaticFiltering=off  FilteringTimeConstant=0.001  PartitionStorageMethod=AS_NEEDED  PartitionMemoryBudget=1024  PartitionMethod=ROBUST
  Terminator : Terminator
  AxTrq : Outport  PortDimensions=[1 4]
  wires:
  Demux/2 -> Simulink-PS Converter6/1
  Demux/3 -> Simulink-PS Converter1/1
  Demux/1 -> Simulink-PS Converter2/1
  Constant1/1 -> Demux/1
  Mux/1 -> Terminator/1
  PS-Simulink Converter1/1 -> Mux/3
  Demux1/3 -> Simulink-PS Converter5/1
  PS-Simulink Converter3/1 -> Mux/4
  Demux/4 -> Simulink-PS Converter3/1
  Demux1/4 -> Simulink-PS Converter4/1
  PS-Simulink Converter2/1 -> Mux/1
  Demux1/1 -> Simulink-PS Converter8/1
  Demux1/2 -> Simulink-PS Converter7/1
  PS-Simulink Converter4/1 -> Mux/2
  ? -> Demux1/1
  Sun Gear Torque/1 -> Gain/1
  Gain/1 -> AxTrq/1
  connections:
  Compound Planetary Gear1/RConn2 -- Ideal Angular Velocity Source/LConn1 -- Solver Configuration1/RConn1 -- Ideal Torque Source1/LConn1 -- Inertia2/LConn1
  Ideal Torque Source1/RConn2 -- Ideal Angular Velocity Source/RConn2 -- Compound Planetary Gear1/RConn1
  Inertia/LConn1 -- Ideal Torque Sensor1/RConn1
  Ideal Torque Sensor1/LConn1 -- Compound Planetary Gear1/LConn1
  PS-Simulink Converter1/LConn1 -- Ideal Torque Sensor1/RConn2
  Simulink-PS Converter5/RConn1 -- Ideal Angular Velocity Source/RConn1
  Ideal Torque Source1/RConn1 -- Simulink-PS Converter1/RConn1
  Compound Planetary Gear3/RConn2 -- Ideal Angular Velocity Source1/LConn1 -- Solver Configuration3/RConn1 -- Ideal Torque Source3/LConn1 -- Inertia3/LConn1
  Ideal Torque Source3/RConn2 -- Ideal Angular Velocity Source1/RConn2 -- Compound Planetary Gear3/RConn1
  Inertia1/LConn1 -- Ideal Torque Sensor3/RConn1
  Ideal Torque Sensor3/LConn1 -- Compound Planetary Gear3/LConn1
  PS-Simulink Converter3/LConn1 -- Ideal Torque Sensor3/RConn2
  Simulink-PS Converter4/RConn1 -- Ideal Angular Velocity Source1/RConn1
  Ideal Torque Source3/RConn1 -- Simulink-PS Converter3/RConn1
  Ideal Torque Source4/RConn2 -- Ideal Angular Velocity Source3/RConn2 -- Compound Planetary Gear4/RConn1
  Ideal Torque Source2/RConn2 -- Ideal Angular Velocity Source2/RConn2 -- Compound Planetary Gear2/RConn1
  Compound Planetary Gear4/RConn2 -- Ideal Angular Velocity Source3/LConn1 -- Solver Configuration4/RConn1 -- Ideal Torque Source4/LConn1 -- Inertia7/LConn1
  Compound Planetary Gear2/RConn2 -- Ideal Angular Velocity Source2/LConn1 -- Solver Configuration2/RConn1 -- Ideal Torque Source2/LConn1 -- Inertia6/LConn1
  Simulink-PS Converter7/RConn1 -- Ideal Angular Velocity Source3/RConn1
  Ideal Torque Source2/RConn1 -- Simulink-PS Converter2/RConn1
  PS-Simulink Converter2/LConn1 -- Ideal Torque Sensor2/RConn2
  Inertia4/LConn1 -- Ideal Torque Sensor2/RConn1
  PS-Simulink Converter4/LConn1 -- Ideal Torque Sensor4/RConn2
  Ideal Torque Source4/RConn1 -- Simulink-PS Converter6/RConn1
  Inertia5/LConn1 -- Ideal Torque Sensor4/RConn1
  Ideal Torque Sensor4/LConn1 -- Compound Planetary Gear4/LConn1
  Simulink-PS Converter8/RConn1 -- Ideal Angular Velocity Source2/RConn1
  Ideal Torque Sensor2/LConn1 -- Compound Planetary Gear2/LConn1
